simulink model "DHM"  (R2022a)
settings: Solver=FixedStepDiscrete  StartTime=0.0  StopTime=10.0  FixedStep=0.01  RelTol=1e-3
libraries: simulink x8, DoorHndDriver x4, DoorHndReq x4, DoorHndPosSts x4
(part 1 of 2)
settings Model: Creator=DELL  LastModifiedBy=DELL
settings DataIOCC: SaveFormat=StructureWithTime
settings OptimizationCC: DefaultParameterBehavior=Inlined  EnhancedBackFolding=on  PassReuseOutputArgsAs=Individual arguments  ZeroExternalMemoryAtStartup=off  ZeroInternalMemoryAtStartup=off  OptimizeBlockOrder=speed  DifferentSizesBufferReuse=on  OptimizationCustomize=off  EfficientTunableParamExpr=on
settings DebuggingCC: ParameterTunabilityLossMsg=error
settings ModelReferenceCC: ModelReferenceNumInstancesAllowed=Single
settings SFSimCC: MATLABDynamicMemAlloc=off
settings RTWCC: Description=AUTOSAR  SystemTargetFile=autosar.tlc  GenCodeOnly=on  TemplateMakefile=ert_default_tmf
settings CodeAppCC: ForceParamTrailComments=on  IgnoreCustomStorageClasses=off  OperatorAnnotations=on  SimulinkDataObjDesc=on  SFDataObjDesc=on  InsertBlockDesc=on
settings STFCustomTargetCC: TargetLangStandard=C99 (ISO)  MultiwordLength=256  ParMdlRefBuildCompliant=on  CompOptLevelCompliant=on  IncludeMdlTerminateFcn=off  CombineOutputUpdateFcns=on  SuppressErrorStatus=on  ERTCustomFileBanners=on  SupportNonFinite=off  SupportComplex=off  SupportContinuousTime=off  SupportNonInlinedSFcns=off  RemoveResetFunc=on  MATLABClassNameForMDSCustomization=Simulink.SoftwareTarget.ERTCustomization  AutosarCompliant=on  GRTInterface=off  UseToolchainInfoCompliant=on  LookupTableObjectStructAxisOrder=2,1,3,4,...  LUTObjectStructOrderEvenSpacing=Size,Table,Breakpoints  SystemTargetFile=autosar.tlc
settings ERTTargetCC: TargetLangStandard=C99 (ISO)  ConcurrentExecutionCompliant=off  IncludeMdlTerminateFcn=off  SuppressErrorStatus=on  SupportNonFinite=off  SupportComplex=off  ModelStepFunctionPrototypeControlCompliant=off  CPPClassGenCompliant=off  AutosarCompliant=on  LookupTableObjectStructAxisOrder=2,1,3,4,...  LUTObjectStructOrderEvenSpacing=Size,Table,Breakpoints  InlinedParameterPlacement=NonHierarchical  ERTCustomFileTemplate=example_file_process.tlc

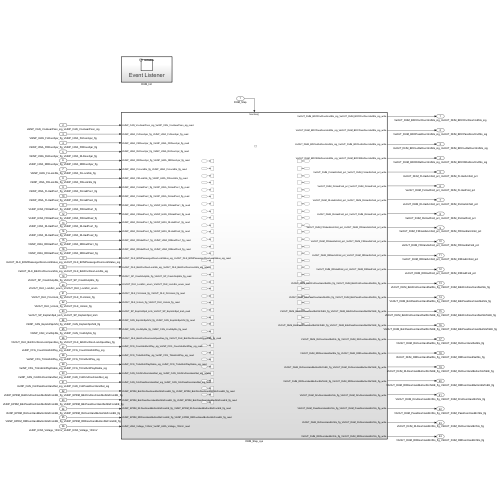
[thumbnail: Simulink's stored preview of the top-level diagram]
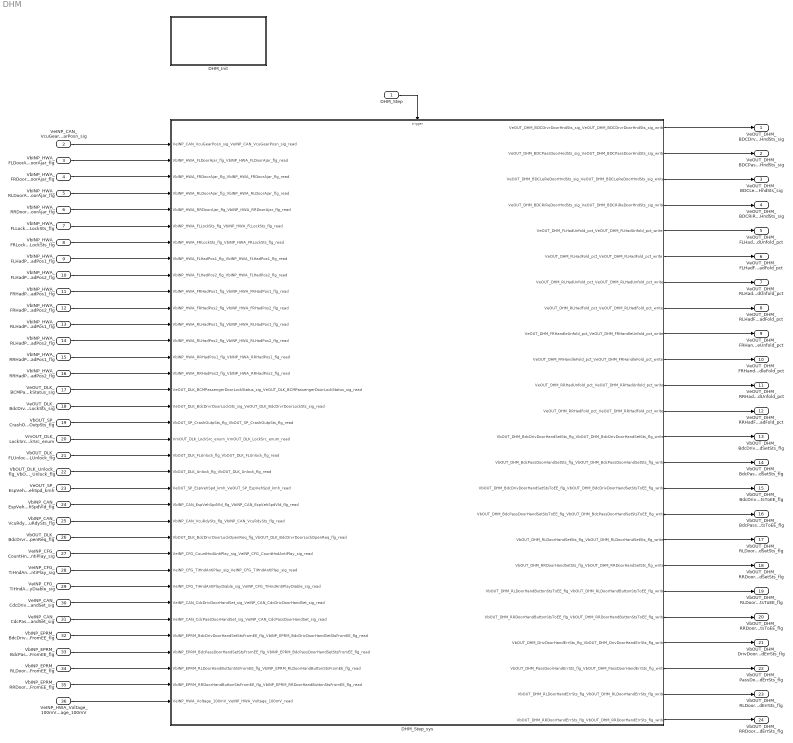
== system DHM ==
  DHM_Step : Inport  SampleTime=0.01  OutputFunctionCall=on
  VeINP_CAN_VcuGearPosn_sig_VeINP_CAN_VcuGearPosn_sig : Inport  Port=2  OutDataTypeStr=UInt8  PortDimensions=1
  VbINP_HWA_FLDoorAjar_flg_VbINP_HWA_FLDoorAjar_flg : Inport  Port=3  OutDataTypeStr=Boolean  PortDimensions=1
  VbINP_HWA_FRDoorAjar_flg_VbINP_HWA_FRDoorAjar_flg : Inport  Port=4  OutDataTypeStr=Boolean  PortDimensions=1
  VbINP_HWA_RLDoorAjar_flg_VbINP_HWA_RLDoorAjar_flg : Inport  Port=5  OutDataTypeStr=Boolean  PortDimensions=1
  VbINP_HWA_RRDoorAjar_flg_VbINP_HWA_RRDoorAjar_flg : Inport  Port=6  OutDataTypeStr=Boolean  PortDimensions=1
  VbINP_HWA_FLLockSts_flg_VbINP_HWA_FLLockSts_flg : Inport  Port=7  OutDataTypeStr=Boolean  PortDimensions=1
  VbINP_HWA_FRLockSts_flg_VbINP_HWA_FRLockSts_flg : Inport  Port=8  OutDataTypeStr=Boolean  PortDimensions=1
  VbINP_HWA_FLHadPos1_flg_VbINP_HWA_FLHadPos1_flg : Inport  Port=9  OutDataTypeStr=Boolean  PortDimensions=1
  VbINP_HWA_FLHadPos2_flg_VbINP_HWA_FLHadPos2_flg : Inport  Port=10  OutDataTypeStr=Boolean  PortDimensions=1
  VbINP_HWA_FRHadPos1_flg_VbINP_HWA_FRHadPos1_flg : Inport  Port=11  OutDataTypeStr=Boolean  PortDimensions=1
  VbINP_HWA_FRHadPos2_flg_VbINP_HWA_FRHadPos2_flg : Inport  Port=12  OutDataTypeStr=Boolean  PortDimensions=1
  VbINP_HWA_RLHadPos1_flg_VbINP_HWA_RLHadPos1_flg : Inport  Port=13  OutDataTypeStr=Boolean  PortDimensions=1
  VbINP_HWA_RLHadPos2_flg_VbINP_HWA_RLHadPos2_flg : Inport  Port=14  OutDataTypeStr=Boolean  PortDimensions=1
  VbINP_HWA_RRHadPos1_flg_VbINP_HWA_RRHadPos1_flg : Inport  Port=15  OutDataTypeStr=Boolean  PortDimensions=1
  VbINP_HWA_RRHadPos2_flg_VbINP_HWA_RRHadPos2_flg : Inport  Port=16  OutDataTypeStr=Boolean  PortDimensions=1
  VeOUT_DLK_BCMPassengerDoorLockStatus_sig_VeOUT_DLK_BCMPassengerDoorLockStatus_sig : Inport  Port=17  OutDataTypeStr=UInt8  PortDimensions=1
  VeOUT_DLK_BdcDrvrDoorLockSts_sig_VeOUT_DLK_BdcDrvrDoorLockSts_sig : Inport  Port=18  OutDataTypeStr=UInt8  PortDimensions=1
  VbOUT_SP_CrashOutpSts_flg_VbOUT_SP_CrashOutpSts_flg : Inport  Port=19  OutDataTypeStr=Boolean  PortDimensions=1
  VmOUT_DLK_LockSrc_enum_VmOUT_DLK_LockSrc_enum : Inport  Port=20  OutDataTypeStr=UInt8  PortDimensions=1
  VbOUT_DLK_FLUnlock_flg_VbOUT_DLK_FLUnlock_flg : Inport  Port=21  OutDataTypeStr=Boolean  PortDimensions=1
  VbOUT_DLK_Unlock_flg_VbOUT_DLK_Unlock_flg : Inport  Port=22  OutDataTypeStr=Boolean  PortDimensions=1
  VeOUT_SP_EspVehSpd_kmh_VeOUT_SP_EspVehSpd_kmh : Inport  Port=23  OutDataTypeStr=UInt8  PortDimensions=1
  VbINP_CAN_EspVehSpdVld_flg_VbINP_CAN_EspVehSpdVld_flg : Inport  Port=24  OutDataTypeStr=Boolean  PortDimensions=1
  VbINP_CAN_VcuRdySts_flg_VbINP_CAN_VcuRdySts_flg : Inport  Port=25  OutDataTypeStr=Boolean  PortDimensions=1
  VbOUT_DLK_BdcDrvrDoorLockOpenReq_flg_VbOUT_DLK_BdcDrvrDoorLockOpenReq_flg : Inport  Port=26  OutDataTypeStr=Boolean  PortDimensions=1
  VeINP_CFG_CountHndAntiPlay_sig_VeINP_CFG_CountHndAntiPlay_sig : Inport  Port=27  OutDataTypeStr=UInt8  PortDimensions=1
  VeINP_CFG_TiHndAntiPlay_sig_VeINP_CFG_TiHndAntiPlay_sig : Inport  Port=28  OutDataTypeStr=UInt8  PortDimensions=1
  VeINP_CFG_TiHndAntiPlayDiable_sig_VeINP_CFG_TiHndAntiPlayDiable_sig : Inport  Port=29  OutDataTypeStr=UInt8  PortDimensions=1
  VeINP_CAN_CdcDrivDoorHandSet_sig_VeINP_CAN_CdcDrivDoorHandSet_sig : Inport  Port=30  OutDataTypeStr=UInt8  PortDimensions=1
  VeINP_CAN_CdcPassDoorHandSet_sig_VeINP_CAN_CdcPassDoorHandSet_sig : Inport  Port=31  OutDataTypeStr=UInt8  PortDimensions=1
  VbINP_EPRM_BdcDrivDoorHandSetStsFromEE_flg_VbINP_EPRM_BdcDrivDoorHandSetStsFromEE_flg : Inport  Port=32  OutDataTypeStr=Boolean  PortDimensions=1
  VbINP_EPRM_BdcPassDoorHandSetStsFromEE_flg_VbINP_EPRM_BdcPassDoorHandSetStsFromEE_flg : Inport  Port=33  OutDataTypeStr=Boolean  PortDimensions=1
  VbINP_EPRM_RLDoorHandButtonStsFromEE_flg_VbINP_EPRM_RLDoorHandButtonStsFromEE_flg : Inport  Port=34  OutDataTypeStr=Boolean  PortDimensions=1
  VbINP_EPRM_RRDoorHandButtonStsFromEE_flg_VbINP_EPRM_RRDoorHandButtonStsFromEE_flg : Inport  Port=35  OutDataTypeStr=Boolean  PortDimensions=1
  VeINP_HWA_Voltage_100mV_VeINP_HWA_Voltage_100mV : Inport  Port=36  OutDataTypeStr=UInt8  PortDimensions=1
  DHM_Init : Subsystem
  DHM_Step_sys : Subsystem
  VeOUT_DHM_BDCDrvrDoorHndSts_sig_VeOUT_DHM_BDCDrvrDoorHndSts_sig : Outport  OutDataTypeStr=UInt8  PortDimensions=1
  VeOUT_DHM_BDCPassDoorHndSts_sig_VeOUT_DHM_BDCPassDoorHndSts_sig : Outport  Port=2  OutDataTypeStr=UInt8  PortDimensions=1
  VeOUT_DHM_BDCLeReDoorHndSts_sig_VeOUT_DHM_BDCLeReDoorHndSts_sig : Outport  Port=3  OutDataTypeStr=UInt8  PortDimensions=1
  VeOUT_DHM_BDCRiReDoorHndSts_sig_VeOUT_DHM_BDCRiReDoorHndSts_sig : Outport  Port=4  OutDataTypeStr=UInt8  PortDimensions=1
  VeOUT_DHM_FLHadUnfold_pct_VeOUT_DHM_FLHadUnfold_pct : Outport  Port=5  OutDataTypeStr=UInt8  PortDimensions=1
  VeOUT_DHM_FLHadFold_pct_VeOUT_DHM_FLHadFold_pct : Outport  Port=6  OutDataTypeStr=UInt8  PortDimensions=1
  VeOUT_DHM_RLHadUnfold_pct_VeOUT_DHM_RLHadUnfold_pct : Outport  Port=7  OutDataTypeStr=UInt8  PortDimensions=1
  VeOUT_DHM_RLHadFold_pct_VeOUT_DHM_RLHadFold_pct : Outport  Port=8  OutDataTypeStr=UInt8  PortDimensions=1
  VeOUT_DHM_FRHandleUnfold_pct_VeOUT_DHM_FRHandleUnfold_pct : Outport  Port=9  OutDataTypeStr=UInt8  PortDimensions=1
  VeOUT_DHM_FRHandleFold_pct_VeOUT_DHM_FRHandleFold_pct : Outport  Port=10  OutDataTypeStr=UInt8  PortDimensions=1
  VeOUT_DHM_RRHadUnfold_pct_VeOUT_DHM_RRHadUnfold_pct : Outport  Port=11  OutDataTypeStr=UInt8  PortDimensions=1
  VeOUT_DHM_RRHadFold_pct_VeOUT_DHM_RRHadFold_pct : Outport  Port=12  OutDataTypeStr=UInt8  PortDimensions=1
  VbOUT_DHM_BdcDrivDoorHandSetSts_flg_VbOUT_DHM_BdcDrivDoorHandSetSts_flg : Outport  Port=13  OutDataTypeStr=Boolean  PortDimensions=1
  VbOUT_DHM_BdcPassDoorHandSetSts_flg_VbOUT_DHM_BdcPassDoorHandSetSts_flg : Outport  Port=14  OutDataTypeStr=Boolean  PortDimensions=1
  VbOUT_DHM_BdcDrivDoorHandSetStsToEE_flg_VbOUT_DHM_BdcDrivDoorHandSetStsToEE_flg : Outport  Port=15  OutDataTypeStr=Boolean  PortDimensions=1
  VbOUT_DHM_BdcPassDoorHandSetStsToEE_flg_VbOUT_DHM_BdcPassDoorHandSetStsToEE_flg : Outport  Port=16  OutDataTypeStr=Boolean  PortDimensions=1
  VbOUT_DHM_RLDoorHandSetSts_flg_VbOUT_DHM_RLDoorHandSetSts_flg : Outport  Port=17  OutDataTypeStr=Boolean  PortDimensions=1
  VbOUT_DHM_RRDoorHandSetSts_flg_VbOUT_DHM_RRDoorHandSetSts_flg : Outport  Port=18  OutDataTypeStr=Boolean  PortDimensions=1
  VbOUT_DHM_RLDoorHandButtonStsToEE_flg_VbOUT_DHM_RLDoorHandButtonStsToEE_flg : Outport  Port=19  OutDataTypeStr=Boolean  PortDimensions=1
  VbOUT_DHM_RRDoorHandButtonStsToEE_flg_VbOUT_DHM_RRDoorHandButtonStsToEE_flg : Outport  Port=20  OutDataTypeStr=Boolean  PortDimensions=1
  VbOUT_DHM_DrivDoorHandErrSts_flg_VbOUT_DHM_DrivDoorHandErrSts_flg : Outport  Port=21  OutDataTypeStr=Boolean  PortDimensions=1
  VbOUT_DHM_PassDoorHandErrSts_flg_VbOUT_DHM_PassDoorHandErrSts_flg : Outport  Port=22  OutDataTypeStr=Boolean  PortDimensions=1
  VbOUT_DHM_RLDoorHandErrSts_flg_VbOUT_DHM_RLDoorHandErrSts_flg : Outport  Port=23  OutDataTypeStr=Boolean  PortDimensions=1
  VbOUT_DHM_RRDoorHandErrSts_flg_VbOUT_DHM_RRDoorHandErrSts_flg : Outport  Port=24  OutDataTypeStr=Boolean  PortDimensions=1
  wires:
  VeINP_CAN_VcuGearPosn_sig_VeINP_CAN_VcuGearPosn_sig/1 -> DHM_Step_sys/1(VeINP_CAN_VcuGearPosn_sig_VeINP_CAN_VcuGearPosn_sig_read)
  VbINP_HWA_FLDoorAjar_flg_VbINP_HWA_FLDoorAjar_flg/1 -> DHM_Step_sys/2(VbINP_HWA_FLDoorAjar_flg_VbINP_HWA_FLDoorAjar_flg_read)
  VbINP_HWA_FRDoorAjar_flg_VbINP_HWA_FRDoorAjar_flg/1 -> DHM_Step_sys/3(VbINP_HWA_FRDoorAjar_flg_VbINP_HWA_FRDoorAjar_flg_read)
  VbINP_HWA_RLDoorAjar_flg_VbINP_HWA_RLDoorAjar_flg/1 -> DHM_Step_sys/4(VbINP_HWA_RLDoorAjar_flg_VbINP_HWA_RLDoorAjar_flg_read)
  VbINP_HWA_RRDoorAjar_flg_VbINP_HWA_RRDoorAjar_flg/1 -> DHM_Step_sys/5(VbINP_HWA_RRDoorAjar_flg_VbINP_HWA_RRDoorAjar_flg_read)
  VbINP_HWA_FLLockSts_flg_VbINP_HWA_FLLockSts_flg/1 -> DHM_Step_sys/6(VbINP_HWA_FLLockSts_flg_VbINP_HWA_FLLockSts_flg_read)
  VbINP_HWA_FRLockSts_flg_VbINP_HWA_FRLockSts_flg/1 -> DHM_Step_sys/7(VbINP_HWA_FRLockSts_flg_VbINP_HWA_FRLockSts_flg_read)
  VbINP_HWA_FLHadPos1_flg_VbINP_HWA_FLHadPos1_flg/1 -> DHM_Step_sys/8(VbINP_HWA_FLHadPos1_flg_VbINP_HWA_FLHadPos1_flg_read)
  VbINP_HWA_FLHadPos2_flg_VbINP_HWA_FLHadPos2_flg/1 -> DHM_Step_sys/9(VbINP_HWA_FLHadPos2_flg_VbINP_HWA_FLHadPos2_flg_read)
  VbINP_HWA_FRHadPos1_flg_VbINP_HWA_FRHadPos1_flg/1 -> DHM_Step_sys/10(VbINP_HWA_FRHadPos1_flg_VbINP_HWA_FRHadPos1_flg_read)
  VbINP_HWA_FRHadPos2_flg_VbINP_HWA_FRHadPos2_flg/1 -> DHM_Step_sys/11(VbINP_HWA_FRHadPos2_flg_VbINP_HWA_FRHadPos2_flg_read)
  VbINP_HWA_RLHadPos1_flg_VbINP_HWA_RLHadPos1_flg/1 -> DHM_Step_sys/12(VbINP_HWA_RLHadPos1_flg_VbINP_HWA_RLHadPos1_flg_read)
  VbINP_HWA_RLHadPos2_flg_VbINP_HWA_RLHadPos2_flg/1 -> DHM_Step_sys/13(VbINP_HWA_RLHadPos2_flg_VbINP_HWA_RLHadPos2_flg_read)
  VbINP_HWA_RRHadPos1_flg_VbINP_HWA_RRHadPos1_flg/1 -> DHM_Step_sys/14(VbINP_HWA_RRHadPos1_flg_VbINP_HWA_RRHadPos1_flg_read)
  VbINP_HWA_RRHadPos2_flg_VbINP_HWA_RRHadPos2_flg/1 -> DHM_Step_sys/15(VbINP_HWA_RRHadPos2_flg_VbINP_HWA_RRHadPos2_flg_read)
  VeOUT_DLK_BCMPassengerDoorLockStatus_sig_VeOUT_DLK_BCMPassengerDoorLockStatus_sig/1 -> DHM_Step_sys/16(VeOUT_DLK_BCMPassengerDoorLockStatus_sig_VeOUT_DLK_BCMPassengerDoorLockStatus_sig_read)
  VeOUT_DLK_BdcDrvrDoorLockSts_sig_VeOUT_DLK_BdcDrvrDoorLockSts_sig/1 -> DHM_Step_sys/17(VeOUT_DLK_BdcDrvrDoorLockSts_sig_VeOUT_DLK_BdcDrvrDoorLockSts_sig_read)
  VbOUT_SP_CrashOutpSts_flg_VbOUT_SP_CrashOutpSts_flg/1 -> DHM_Step_sys/18(VbOUT_SP_CrashOutpSts_flg_VbOUT_SP_CrashOutpSts_flg_read)
  VmOUT_DLK_LockSrc_enum_VmOUT_DLK_LockSrc_enum/1 -> DHM_Step_sys/19(VmOUT_DLK_LockSrc_enum_VmOUT_DLK_LockSrc_enum_read)
  VbOUT_DLK_FLUnlock_flg_VbOUT_DLK_FLUnlock_flg/1 -> DHM_Step_sys/20(VbOUT_DLK_FLUnlock_flg_VbOUT_DLK_FLUnlock_flg_read)
  VbOUT_DLK_Unlock_flg_VbOUT_DLK_Unlock_flg/1 -> DHM_Step_sys/21(VbOUT_DLK_Unlock_flg_VbOUT_DLK_Unlock_flg_read)
  VeOUT_SP_EspVehSpd_kmh_VeOUT_SP_EspVehSpd_kmh/1 -> DHM_Step_sys/22(VeOUT_SP_EspVehSpd_kmh_VeOUT_SP_EspVehSpd_kmh_read)
  VbINP_CAN_EspVehSpdVld_flg_VbINP_CAN_EspVehSpdVld_flg/1 -> DHM_Step_sys/23(VbINP_CAN_EspVehSpdVld_flg_VbINP_CAN_EspVehSpdVld_flg_read)
  VbINP_CAN_VcuRdySts_flg_VbINP_CAN_VcuRdySts_flg/1 -> DHM_Step_sys/24(VbINP_CAN_VcuRdySts_flg_VbINP_CAN_VcuRdySts_flg_read)
  VbOUT_DLK_BdcDrvrDoorLockOpenReq_flg_VbOUT_DLK_BdcDrvrDoorLockOpenReq_flg/1 -> DHM_Step_sys/25(VbOUT_DLK_BdcDrvrDoorLockOpenReq_flg_VbOUT_DLK_BdcDrvrDoorLockOpenReq_flg_read)
  VeINP_CFG_CountHndAntiPlay_sig_VeINP_CFG_CountHndAntiPlay_sig/1 -> DHM_Step_sys/26(VeINP_CFG_CountHndAntiPlay_sig_VeINP_CFG_CountHndAntiPlay_sig_read)
  VeINP_CFG_TiHndAntiPlay_sig_VeINP_CFG_TiHndAntiPlay_sig/1 -> DHM_Step_sys/27(VeINP_CFG_TiHndAntiPlay_sig_VeINP_CFG_TiHndAntiPlay_sig_read)
  VeINP_CFG_TiHndAntiPlayDiable_sig_VeINP_CFG_TiHndAntiPlayDiable_sig/1 -> DHM_Step_sys/28(VeINP_CFG_TiHndAntiPlayDiable_sig_VeINP_CFG_TiHndAntiPlayDiable_sig_read)
  VeINP_CAN_CdcDrivDoorHandSet_sig_VeINP_CAN_CdcDrivDoorHandSet_sig/1 -> DHM_Step_sys/29(VeINP_CAN_CdcDrivDoorHandSet_sig_VeINP_CAN_CdcDrivDoorHandSet_sig_read)
  VeINP_CAN_CdcPassDoorHandSet_sig_VeINP_CAN_CdcPassDoorHandSet_sig/1 -> DHM_Step_sys/30(VeINP_CAN_CdcPassDoorHandSet_sig_VeINP_CAN_CdcPassDoorHandSet_sig_read)
  VbINP_EPRM_BdcDrivDoorHandSetStsFromEE_flg_VbINP_EPRM_BdcDrivDoorHandSetStsFromEE_flg/1 -> DHM_Step_sys/31(VbINP_EPRM_BdcDrivDoorHandSetStsFromEE_flg_VbINP_EPRM_BdcDrivDoorHandSetStsFromEE_flg_read)
  VbINP_EPRM_BdcPassDoorHandSetStsFromEE_flg_VbINP_EPRM_BdcPassDoorHandSetStsFromEE_flg/1 -> DHM_Step_sys/32(VbINP_EPRM_BdcPassDoorHandSetStsFromEE_flg_VbINP_EPRM_BdcPassDoorHandSetStsFromEE_flg_read)
  VbINP_EPRM_RLDoorHandButtonStsFromEE_flg_VbINP_EPRM_RLDoorHandButtonStsFromEE_flg/1 -> DHM_Step_sys/33(VbINP_EPRM_RLDoorHandButtonStsFromEE_flg_VbINP_EPRM_RLDoorHandButtonStsFromEE_flg_read)
  VbINP_EPRM_RRDoorHandButtonStsFromEE_flg_VbINP_EPRM_RRDoorHandButtonStsFromEE_flg/1 -> DHM_Step_sys/34(VbINP_EPRM_RRDoorHandButtonStsFromEE_flg_VbINP_EPRM_RRDoorHandButtonStsFromEE_flg_read)
  VeINP_HWA_Voltage_100mV_VeINP_HWA_Voltage_100mV/1 -> DHM_Step_sys/35(VeINP_HWA_Voltage_100mV_VeINP_HWA_Voltage_100mV_read)
  DHM_Step_sys/1(VeOUT_DHM_BDCDrvrDoorHndSts_sig_VeOUT_DHM_BDCDrvrDoorHndSts_sig_write) -> VeOUT_DHM_BDCDrvrDoorHndSts_sig_VeOUT_DHM_BDCDrvrDoorHndSts_sig/1
  DHM_Step_sys/2(VeOUT_DHM_BDCPassDoorHndSts_sig_VeOUT_DHM_BDCPassDoorHndSts_sig_write) -> VeOUT_DHM_BDCPassDoorHndSts_sig_VeOUT_DHM_BDCPassDoorHndSts_sig/1
  DHM_Step_sys/3(VeOUT_DHM_BDCLeReDoorHndSts_sig_VeOUT_DHM_BDCLeReDoorHndSts_sig_write) -> VeOUT_DHM_BDCLeReDoorHndSts_sig_VeOUT_DHM_BDCLeReDoorHndSts_sig/1
  DHM_Step_sys/4(VeOUT_DHM_BDCRiReDoorHndSts_sig_VeOUT_DHM_BDCRiReDoorHndSts_sig_write) -> VeOUT_DHM_BDCRiReDoorHndSts_sig_VeOUT_DHM_BDCRiReDoorHndSts_sig/1
  DHM_Step_sys/5(VeOUT_DHM_FLHadUnfold_pct_VeOUT_DHM_FLHadUnfold_pct_write) -> VeOUT_DHM_FLHadUnfold_pct_VeOUT_DHM_FLHadUnfold_pct/1
  DHM_Step_sys/6(VeOUT_DHM_FLHadFold_pct_VeOUT_DHM_FLHadFold_pct_write) -> VeOUT_DHM_FLHadFold_pct_VeOUT_DHM_FLHadFold_pct/1
  DHM_Step_sys/7(VeOUT_DHM_RLHadUnfold_pct_VeOUT_DHM_RLHadUnfold_pct_write) -> VeOUT_DHM_RLHadUnfold_pct_VeOUT_DHM_RLHadUnfold_pct/1
  DHM_Step_sys/8(VeOUT_DHM_RLHadFold_pct_VeOUT_DHM_RLHadFold_pct_write) -> VeOUT_DHM_RLHadFold_pct_VeOUT_DHM_RLHadFold_pct/1
  DHM_Step_sys/9(VeOUT_DHM_FRHandleUnfold_pct_VeOUT_DHM_FRHandleUnfold_pct_write) -> VeOUT_DHM_FRHandleUnfold_pct_VeOUT_DHM_FRHandleUnfold_pct/1
  DHM_Step_sys/10(VeOUT_DHM_FRHandleFold_pct_VeOUT_DHM_FRHandleFold_pct_write) -> VeOUT_DHM_FRHandleFold_pct_VeOUT_DHM_FRHandleFold_pct/1
  DHM_Step_sys/11(VeOUT_DHM_RRHadUnfold_pct_VeOUT_DHM_RRHadUnfold_pct_write) -> VeOUT_DHM_RRHadUnfold_pct_VeOUT_DHM_RRHadUnfold_pct/1
  DHM_Step_sys/12(VeOUT_DHM_RRHadFold_pct_VeOUT_DHM_RRHadFold_pct_write) -> VeOUT_DHM_RRHadFold_pct_VeOUT_DHM_RRHadFold_pct/1
  DHM_Step_sys/13(VbOUT_DHM_BdcDrivDoorHandSetSts_flg_VbOUT_DHM_BdcDrivDoorHandSetSts_flg_write) -> VbOUT_DHM_BdcDrivDoorHandSetSts_flg_VbOUT_DHM_BdcDrivDoorHandSetSts_flg/1
  DHM_Step_sys/14(VbOUT_DHM_BdcPassDoorHandSetSts_flg_VbOUT_DHM_BdcPassDoorHandSetSts_flg_write) -> VbOUT_DHM_BdcPassDoorHandSetSts_flg_VbOUT_DHM_BdcPassDoorHandSetSts_flg/1
  DHM_Step_sys/15(VbOUT_DHM_BdcDrivDoorHandSetStsToEE_flg_VbOUT_DHM_BdcDrivDoorHandSetStsToEE_flg_write) -> VbOUT_DHM_BdcDrivDoorHandSetStsToEE_flg_VbOUT_DHM_BdcDrivDoorHandSetStsToEE_flg/1
  DHM_Step_sys/16(VbOUT_DHM_BdcPassDoorHandSetStsToEE_flg_VbOUT_DHM_BdcPassDoorHandSetStsToEE_flg_write) -> VbOUT_DHM_BdcPassDoorHandSetStsToEE_flg_VbOUT_DHM_BdcPassDoorHandSetStsToEE_flg/1
  DHM_Step_sys/17(VbOUT_DHM_RLDoorHandSetSts_flg_VbOUT_DHM_RLDoorHandSetSts_flg_write) -> VbOUT_DHM_RLDoorHandSetSts_flg_VbOUT_DHM_RLDoorHandSetSts_flg/1
  DHM_Step_sys/18(VbOUT_DHM_RRDoorHandSetSts_flg_VbOUT_DHM_RRDoorHandSetSts_flg_write) -> VbOUT_DHM_RRDoorHandSetSts_flg_VbOUT_DHM_RRDoorHandSetSts_flg/1
  DHM_Step_sys/19(VbOUT_DHM_RLDoorHandButtonStsToEE_flg_VbOUT_DHM_RLDoorHandButtonStsToEE_flg_write) -> VbOUT_DHM_RLDoorHandButtonStsToEE_flg_VbOUT_DHM_RLDoorHandButtonStsToEE_flg/1
  DHM_Step_sys/20(VbOUT_DHM_RRDoorHandButtonStsToEE_flg_VbOUT_DHM_RRDoorHandButtonStsToEE_flg_write) -> VbOUT_DHM_RRDoorHandButtonStsToEE_flg_VbOUT_DHM_RRDoorHandButtonStsToEE_flg/1
  DHM_Step_sys/21(VbOUT_DHM_DrivDoorHandErrSts_flg_VbOUT_DHM_DrivDoorHandErrSts_flg_write) -> VbOUT_DHM_DrivDoorHandErrSts_flg_VbOUT_DHM_DrivDoorHandErrSts_flg/1
  DHM_Step_sys/22(VbOUT_DHM_PassDoorHandErrSts_flg_VbOUT_DHM_PassDoorHandErrSts_flg_write) -> VbOUT_DHM_PassDoorHandErrSts_flg_VbOUT_DHM_PassDoorHandErrSts_flg/1
  DHM_Step_sys/23(VbOUT_DHM_RLDoorHandErrSts_flg_VbOUT_DHM_RLDoorHandErrSts_flg_write) -> VbOUT_DHM_RLDoorHandErrSts_flg_VbOUT_DHM_RLDoorHandErrSts_flg/1
  DHM_Step_sys/24(VbOUT_DHM_RRDoorHandErrSts_flg_VbOUT_DHM_RRDoorHandErrSts_flg_write) -> VbOUT_DHM_RRDoorHandErrSts_flg_VbOUT_DHM_RRDoorHandErrSts_flg/1
  DHM_Step/1 -> DHM_Step_sys/Trigger

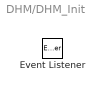
== system DHM/DHM_Init ==
  Event Listener : EventListener  EventName=reset

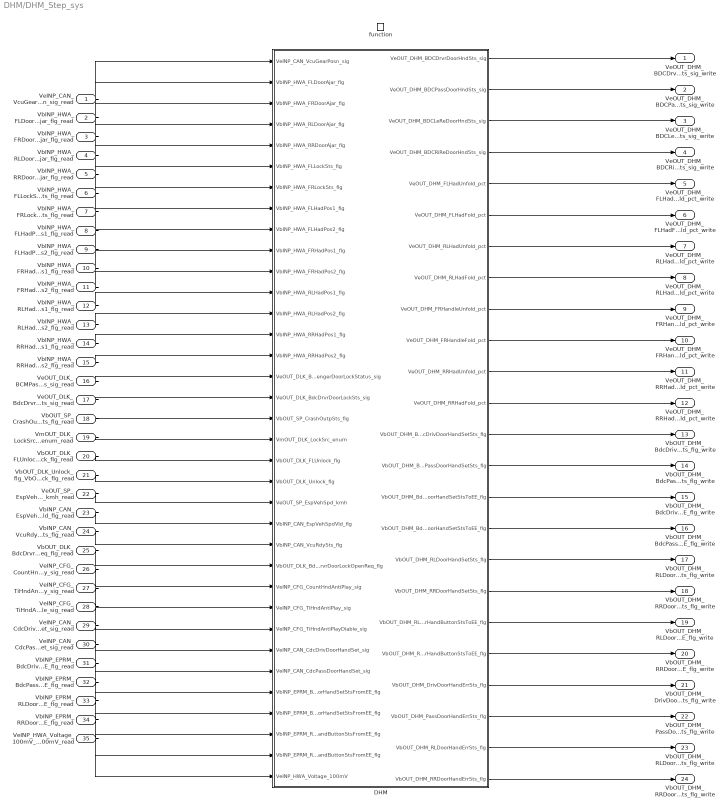
== system DHM/DHM_Step_sys ==
  VeINP_CAN_VcuGearPosn_sig_VeINP_CAN_VcuGearPosn_sig_read : Inport
  VbINP_HWA_FLDoorAjar_flg_VbINP_HWA_FLDoorAjar_flg_read : Inport  Port=2
  VbINP_HWA_FRDoorAjar_flg_VbINP_HWA_FRDoorAjar_flg_read : Inport  Port=3
  VbINP_HWA_RLDoorAjar_flg_VbINP_HWA_RLDoorAjar_flg_read : Inport  Port=4
  VbINP_HWA_RRDoorAjar_flg_VbINP_HWA_RRDoorAjar_flg_read : Inport  Port=5
  VbINP_HWA_FLLockSts_flg_VbINP_HWA_FLLockSts_flg_read : Inport  Port=6
  VbINP_HWA_FRLockSts_flg_VbINP_HWA_FRLockSts_flg_read : Inport  Port=7
  VbINP_HWA_FLHadPos1_flg_VbINP_HWA_FLHadPos1_flg_read : Inport  Port=8
  VbINP_HWA_FLHadPos2_flg_VbINP_HWA_FLHadPos2_flg_read : Inport  Port=9
  VbINP_HWA_FRHadPos1_flg_VbINP_HWA_FRHadPos1_flg_read : Inport  Port=10
  VbINP_HWA_FRHadPos2_flg_VbINP_HWA_FRHadPos2_flg_read : Inport  Port=11
  VbINP_HWA_RLHadPos1_flg_VbINP_HWA_RLHadPos1_flg_read : Inport  Port=12
  VbINP_HWA_RLHadPos2_flg_VbINP_HWA_RLHadPos2_flg_read : Inport  Port=13
  VbINP_HWA_RRHadPos1_flg_VbINP_HWA_RRHadPos1_flg_read : Inport  Port=14
  VbINP_HWA_RRHadPos2_flg_VbINP_HWA_RRHadPos2_flg_read : Inport  Port=15
  VeOUT_DLK_BCMPassengerDoorLockStatus_sig_VeOUT_DLK_BCMPassengerDoorLockStatus_sig_read : Inport  Port=16
  VeOUT_DLK_BdcDrvrDoorLockSts_sig_VeOUT_DLK_BdcDrvrDoorLockSts_sig_read : Inport  Port=17
  VbOUT_SP_CrashOutpSts_flg_VbOUT_SP_CrashOutpSts_flg_read : Inport  Port=18
  VmOUT_DLK_LockSrc_enum_VmOUT_DLK_LockSrc_enum_read : Inport  Port=19
  VbOUT_DLK_FLUnlock_flg_VbOUT_DLK_FLUnlock_flg_read : Inport  Port=20
  VbOUT_DLK_Unlock_flg_VbOUT_DLK_Unlock_flg_read : Inport  Port=21
  VeOUT_SP_EspVehSpd_kmh_VeOUT_SP_EspVehSpd_kmh_read : Inport  Port=22
  VbINP_CAN_EspVehSpdVld_flg_VbINP_CAN_EspVehSpdVld_flg_read : Inport  Port=23
  VbINP_CAN_VcuRdySts_flg_VbINP_CAN_VcuRdySts_flg_read : Inport  Port=24
  VbOUT_DLK_BdcDrvrDoorLockOpenReq_flg_VbOUT_DLK_BdcDrvrDoorLockOpenReq_flg_read : Inport  Port=25
  VeINP_CFG_CountHndAntiPlay_sig_VeINP_CFG_CountHndAntiPlay_sig_read : Inport  Port=26
  VeINP_CFG_TiHndAntiPlay_sig_VeINP_CFG_TiHndAntiPlay_sig_read : Inport  Port=27
  VeINP_CFG_TiHndAntiPlayDiable_sig_VeINP_CFG_TiHndAntiPlayDiable_sig_read : Inport  Port=28
  VeINP_CAN_CdcDrivDoorHandSet_sig_VeINP_CAN_CdcDrivDoorHandSet_sig_read : Inport  Port=29
  VeINP_CAN_CdcPassDoorHandSet_sig_VeINP_CAN_CdcPassDoorHandSet_sig_read : Inport  Port=30
  VbINP_EPRM_BdcDrivDoorHandSetStsFromEE_flg_VbINP_EPRM_BdcDrivDoorHandSetStsFromEE_flg_read : Inport  Port=31
  VbINP_EPRM_BdcPassDoorHandSetStsFromEE_flg_VbINP_EPRM_BdcPassDoorHandSetStsFromEE_flg_read : Inport  Port=32
  VbINP_EPRM_RLDoorHandButtonStsFromEE_flg_VbINP_EPRM_RLDoorHandButtonStsFromEE_flg_read : Inport  Port=33
  VbINP_EPRM_RRDoorHandButtonStsFromEE_flg_VbINP_EPRM_RRDoorHandButtonStsFromEE_flg_read : Inport  Port=34
  VeINP_HWA_Voltage_100mV_VeINP_HWA_Voltage_100mV_read : Inport  Port=35
  function : TriggerPort  TriggerType=function-call  VariantControl=(inherit)  SampleTimeType=periodic  SampleTime=-1
  DHM : Subsystem
  VeOUT_DHM_BDCDrvrDoorHndSts_sig_VeOUT_DHM_BDCDrvrDoorHndSts_sig_write : Outport
      settings: EnsureOutportIsVirtual=on
  VeOUT_DHM_BDCPassDoorHndSts_sig_VeOUT_DHM_BDCPassDoorHndSts_sig_write : Outport  Port=2
      settings: EnsureOutportIsVirtual=on
  VeOUT_DHM_BDCLeReDoorHndSts_sig_VeOUT_DHM_BDCLeReDoorHndSts_sig_write : Outport  Port=3
      settings: EnsureOutportIsVirtual=on
  VeOUT_DHM_BDCRiReDoorHndSts_sig_VeOUT_DHM_BDCRiReDoorHndSts_sig_write : Outport  Port=4
      settings: EnsureOutportIsVirtual=on
  VeOUT_DHM_FLHadUnfold_pct_VeOUT_DHM_FLHadUnfold_pct_write : Outport  Port=5
      settings: EnsureOutportIsVirtual=on
  VeOUT_DHM_FLHadFold_pct_VeOUT_DHM_FLHadFold_pct_write : Outport  Port=6
      settings: EnsureOutportIsVirtual=on
  VeOUT_DHM_RLHadUnfold_pct_VeOUT_DHM_RLHadUnfold_pct_write : Outport  Port=7
      settings: EnsureOutportIsVirtual=on
  VeOUT_DHM_RLHadFold_pct_VeOUT_DHM_RLHadFold_pct_write : Outport  Port=8
      settings: EnsureOutportIsVirtual=on
  VeOUT_DHM_FRHandleUnfold_pct_VeOUT_DHM_FRHandleUnfold_pct_write : Outport  Port=9
      settings: EnsureOutportIsVirtual=on
  VeOUT_DHM_FRHandleFold_pct_VeOUT_DHM_FRHandleFold_pct_write : Outport  Port=10
      settings: EnsureOutportIsVirtual=on
  VeOUT_DHM_RRHadUnfold_pct_VeOUT_DHM_RRHadUnfold_pct_write : Outport  Port=11
      settings: EnsureOutportIsVirtual=on
  VeOUT_DHM_RRHadFold_pct_VeOUT_DHM_RRHadFold_pct_write : Outport  Port=12
      settings: EnsureOutportIsVirtual=on
  VbOUT_DHM_BdcDrivDoorHandSetSts_flg_VbOUT_DHM_BdcDrivDoorHandSetSts_flg_write : Outport  Port=13
      settings: EnsureOutportIsVirtual=on
  VbOUT_DHM_BdcPassDoorHandSetSts_flg_VbOUT_DHM_BdcPassDoorHandSetSts_flg_write : Outport  Port=14
      settings: EnsureOutportIsVirtual=on
  VbOUT_DHM_BdcDrivDoorHandSetStsToEE_flg_VbOUT_DHM_BdcDrivDoorHandSetStsToEE_flg_write : Outport  Port=15
      settings: EnsureOutportIsVirtual=on
  VbOUT_DHM_BdcPassDoorHandSetStsToEE_flg_VbOUT_DHM_BdcPassDoorHandSetStsToEE_flg_write : Outport  Port=16
      settings: EnsureOutportIsVirtual=on
  VbOUT_DHM_RLDoorHandSetSts_flg_VbOUT_DHM_RLDoorHandSetSts_flg_write : Outport  Port=17
      settings: EnsureOutportIsVirtual=on
  VbOUT_DHM_RRDoorHandSetSts_flg_VbOUT_DHM_RRDoorHandSetSts_flg_write : Outport  Port=18
      settings: EnsureOutportIsVirtual=on
  VbOUT_DHM_RLDoorHandButtonStsToEE_flg_VbOUT_DHM_RLDoorHandButtonStsToEE_flg_write : Outport  Port=19
      settings: EnsureOutportIsVirtual=on
  VbOUT_DHM_RRDoorHandButtonStsToEE_flg_VbOUT_DHM_RRDoorHandButtonStsToEE_flg_write : Outport  Port=20
      settings: EnsureOutportIsVirtual=on
  VbOUT_DHM_DrivDoorHandErrSts_flg_VbOUT_DHM_DrivDoorHandErrSts_flg_write : Outport  Port=21
      settings: EnsureOutportIsVirtual=on
  VbOUT_DHM_PassDoorHandErrSts_flg_VbOUT_DHM_PassDoorHandErrSts_flg_write : Outport  Port=22
      settings: EnsureOutportIsVirtual=on
  VbOUT_DHM_RLDoorHandErrSts_flg_VbOUT_DHM_RLDoorHandErrSts_flg_write : Outport  Port=23
      settings: EnsureOutportIsVirtual=on
  VbOUT_DHM_RRDoorHandErrSts_flg_VbOUT_DHM_RRDoorHandErrSts_flg_write : Outport  Port=24
      settings: EnsureOutportIsVirtual=on
  wires:
  DHM/4(VeOUT_DHM_BDCRiReDoorHndSts_sig) -> VeOUT_DHM_BDCRiReDoorHndSts_sig_VeOUT_DHM_BDCRiReDoorHndSts_sig_write/1
  DHM/3(VeOUT_DHM_BDCLeReDoorHndSts_sig) -> VeOUT_DHM_BDCLeReDoorHndSts_sig_VeOUT_DHM_BDCLeReDoorHndSts_sig_write/1
  DHM/5(VeOUT_DHM_FLHadUnfold_pct) -> VeOUT_DHM_FLHadUnfold_pct_VeOUT_DHM_FLHadUnfold_pct_write/1
  DHM/2(VeOUT_DHM_BDCPassDoorHndSts_sig) -> VeOUT_DHM_BDCPassDoorHndSts_sig_VeOUT_DHM_BDCPassDoorHndSts_sig_write/1
  DHM/1(VeOUT_DHM_BDCDrvrDoorHndSts_sig) -> VeOUT_DHM_BDCDrvrDoorHndSts_sig_VeOUT_DHM_BDCDrvrDoorHndSts_sig_write/1
  DHM/6(VeOUT_DHM_FLHadFold_pct) -> VeOUT_DHM_FLHadFold_pct_VeOUT_DHM_FLHadFold_pct_write/1
  DHM/7(VeOUT_DHM_RLHadUnfold_pct) -> VeOUT_DHM_RLHadUnfold_pct_VeOUT_DHM_RLHadUnfold_pct_write/1
  DHM/8(VeOUT_DHM_RLHadFold_pct) -> VeOUT_DHM_RLHadFold_pct_VeOUT_DHM_RLHadFold_pct_write/1
  DHM/9(VeOUT_DHM_FRHandleUnfold_pct) -> VeOUT_DHM_FRHandleUnfold_pct_VeOUT_DHM_FRHandleUnfold_pct_write/1
  DHM/10(VeOUT_DHM_FRHandleFold_pct) -> VeOUT_DHM_FRHandleFold_pct_VeOUT_DHM_FRHandleFold_pct_write/1
  DHM/11(VeOUT_DHM_RRHadUnfold_pct) -> VeOUT_DHM_RRHadUnfold_pct_VeOUT_DHM_RRHadUnfold_pct_write/1
  DHM/12(VeOUT_DHM_RRHadFold_pct) -> VeOUT_DHM_RRHadFold_pct_VeOUT_DHM_RRHadFold_pct_write/1
  DHM/13(VbOUT_DHM_BdcDrivDoorHandSetSts_flg) -> VbOUT_DHM_BdcDrivDoorHandSetSts_flg_VbOUT_DHM_BdcDrivDoorHandSetSts_flg_write/1
  DHM/14(VbOUT_DHM_BdcPassDoorHandSetSts_flg) -> VbOUT_DHM_BdcPassDoorHandSetSts_flg_VbOUT_DHM_BdcPassDoorHandSetSts_flg_write/1
  DHM/15(VbOUT_DHM_BdcDrivDoorHandSetStsToEE_flg) -> VbOUT_DHM_BdcDrivDoorHandSetStsToEE_flg_VbOUT_DHM_BdcDrivDoorHandSetStsToEE_flg_write/1
  DHM/16(VbOUT_DHM_BdcPassDoorHandSetStsToEE_flg) -> VbOUT_DHM_BdcPassDoorHandSetStsToEE_flg_VbOUT_DHM_BdcPassDoorHandSetStsToEE_flg_write/1
  DHM/17("VbOUT_DHM_RLDoorHandSetSts_flg ") -> VbOUT_DHM_RLDoorHandSetSts_flg_VbOUT_DHM_RLDoorHandSetSts_flg_write/1
  DHM/18("VbOUT_DHM_RRDoorHandSetSts_flg ") -> VbOUT_DHM_RRDoorHandSetSts_flg_VbOUT_DHM_RRDoorHandSetSts_flg_write/1
  DHM/19("VbOUT_DHM_RLDoorHandButtonStsToEE_flg ") -> VbOUT_DHM_RLDoorHandButtonStsToEE_flg_VbOUT_DHM_RLDoorHandButtonStsToEE_flg_write/1
  DHM/20("VbOUT_DHM_RRDoorHandButtonStsToEE_flg ") -> VbOUT_DHM_RRDoorHandButtonStsToEE_flg_VbOUT_DHM_RRDoorHandButtonStsToEE_flg_write/1
  DHM/21(VbOUT_DHM_DrivDoorHandErrSts_flg) -> VbOUT_DHM_DrivDoorHandErrSts_flg_VbOUT_DHM_DrivDoorHandErrSts_flg_write/1
  DHM/22(VbOUT_DHM_PassDoorHandErrSts_flg) -> VbOUT_DHM_PassDoorHandErrSts_flg_VbOUT_DHM_PassDoorHandErrSts_flg_write/1
  DHM/23(VbOUT_DHM_RLDoorHandErrSts_flg) -> VbOUT_DHM_RLDoorHandErrSts_flg_VbOUT_DHM_RLDoorHandErrSts_flg_write/1
  DHM/24(VbOUT_DHM_RRDoorHandErrSts_flg) -> VbOUT_DHM_RRDoorHandErrSts_flg_VbOUT_DHM_RRDoorHandErrSts_flg_write/1
  VbINP_HWA_RRDoorAjar_flg_VbINP_HWA_RRDoorAjar_flg_read/1 -> DHM/5(VbINP_HWA_RRDoorAjar_flg)
  VbINP_HWA_FLLockSts_flg_VbINP_HWA_FLLockSts_flg_read/1 -> DHM/6(VbINP_HWA_FLLockSts_flg)
  VbINP_HWA_RLDoorAjar_flg_VbINP_HWA_RLDoorAjar_flg_read/1 -> DHM/4(VbINP_HWA_RLDoorAjar_flg)
  VbINP_HWA_FRDoorAjar_flg_VbINP_HWA_FRDoorAjar_flg_read/1 -> DHM/3(VbINP_HWA_FRDoorAjar_flg)
  VbINP_HWA_FRLockSts_flg_VbINP_HWA_FRLockSts_flg_read/1 -> DHM/7(VbINP_HWA_FRLockSts_flg)
  VbINP_HWA_FLDoorAjar_flg_VbINP_HWA_FLDoorAjar_flg_read/1 -> DHM/2(VbINP_HWA_FLDoorAjar_flg)
  VbINP_HWA_FLHadPos1_flg_VbINP_HWA_FLHadPos1_flg_read/1 -> DHM/8(VbINP_HWA_FLHadPos1_flg)
  VbINP_HWA_FLHadPos2_flg_VbINP_HWA_FLHadPos2_flg_read/1 -> DHM/9(VbINP_HWA_FLHadPos2_flg)
  VeINP_CAN_VcuGearPosn_sig_VeINP_CAN_VcuGearPosn_sig_read/1 -> DHM/1(VeINP_CAN_VcuGearPosn_sig)
  VbINP_HWA_FRHadPos1_flg_VbINP_HWA_FRHadPos1_flg_read/1 -> DHM/10(VbINP_HWA_FRHadPos1_flg)
  VbINP_HWA_FRHadPos2_flg_VbINP_HWA_FRHadPos2_flg_read/1 -> DHM/11(VbINP_HWA_FRHadPos2_flg)
  VbINP_HWA_RLHadPos1_flg_VbINP_HWA_RLHadPos1_flg_read/1 -> DHM/12(VbINP_HWA_RLHadPos1_flg)
  VbINP_HWA_RLHadPos2_flg_VbINP_HWA_RLHadPos2_flg_read/1 -> DHM/13(VbINP_HWA_RLHadPos2_flg)
  VbINP_HWA_RRHadPos1_flg_VbINP_HWA_RRHadPos1_flg_read/1 -> DHM/14(VbINP_HWA_RRHadPos1_flg)
  VbINP_HWA_RRHadPos2_flg_VbINP_HWA_RRHadPos2_flg_read/1 -> DHM/15(VbINP_HWA_RRHadPos2_flg)
  VeOUT_DLK_BCMPassengerDoorLockStatus_sig_VeOUT_DLK_BCMPassengerDoorLockStatus_sig_read/1 -> DHM/16(VeOUT_DLK_BCMPassengerDoorLockStatus_sig)
  VeOUT_DLK_BdcDrvrDoorLockSts_sig_VeOUT_DLK_BdcDrvrDoorLockSts_sig_read/1 -> DHM/17(VeOUT_DLK_BdcDrvrDoorLockSts_sig)
  VbOUT_SP_CrashOutpSts_flg_VbOUT_SP_CrashOutpSts_flg_read/1 -> DHM/18(VbOUT_SP_CrashOutpSts_flg)
  VmOUT_DLK_LockSrc_enum_VmOUT_DLK_LockSrc_enum_read/1 -> DHM/19(VmOUT_DLK_LockSrc_enum)
  VbOUT_DLK_FLUnlock_flg_VbOUT_DLK_FLUnlock_flg_read/1 -> DHM/20(VbOUT_DLK_FLUnlock_flg)
  VbOUT_DLK_Unlock_flg_VbOUT_DLK_Unlock_flg_read/1 -> DHM/21(VbOUT_DLK_Unlock_flg)
  VeOUT_SP_EspVehSpd_kmh_VeOUT_SP_EspVehSpd_kmh_read/1 -> DHM/22(VeOUT_SP_EspVehSpd_kmh)
  VbINP_CAN_EspVehSpdVld_flg_VbINP_CAN_EspVehSpdVld_flg_read/1 -> DHM/23(VbINP_CAN_EspVehSpdVld_flg)
  VbINP_CAN_VcuRdySts_flg_VbINP_CAN_VcuRdySts_flg_read/1 -> DHM/24(VbINP_CAN_VcuRdySts_flg)
  VbOUT_DLK_BdcDrvrDoorLockOpenReq_flg_VbOUT_DLK_BdcDrvrDoorLockOpenReq_flg_read/1 -> DHM/25(VbOUT_DLK_BdcDrvrDoorLockOpenReq_flg)
  VeINP_CFG_CountHndAntiPlay_sig_VeINP_CFG_CountHndAntiPlay_sig_read/1 -> DHM/26(VeINP_CFG_CountHndAntiPlay_sig)
  VeINP_CFG_TiHndAntiPlay_sig_VeINP_CFG_TiHndAntiPlay_sig_read/1 -> DHM/27(VeINP_CFG_TiHndAntiPlay_sig)
  VeINP_CFG_TiHndAntiPlayDiable_sig_VeINP_CFG_TiHndAntiPlayDiable_sig_read/1 -> DHM/28(VeINP_CFG_TiHndAntiPlayDiable_sig)
  VeINP_CAN_CdcDrivDoorHandSet_sig_VeINP_CAN_CdcDrivDoorHandSet_sig_read/1 -> DHM/29(VeINP_CAN_CdcDrivDoorHandSet_sig)
  VeINP_CAN_CdcPassDoorHandSet_sig_VeINP_CAN_CdcPassDoorHandSet_sig_read/1 -> DHM/30(VeINP_CAN_CdcPassDoorHandSet_sig)
  VbINP_EPRM_BdcDrivDoorHandSetStsFromEE_flg_VbINP_EPRM_BdcDrivDoorHandSetStsFromEE_flg_read/1 -> DHM/31(VbINP_EPRM_BdcDrivDoorHandSetStsFromEE_flg)
  VbINP_EPRM_BdcPassDoorHandSetStsFromEE_flg_VbINP_EPRM_BdcPassDoorHandSetStsFromEE_flg_read/1 -> DHM/32(VbINP_EPRM_BdcPassDoorHandSetStsFromEE_flg)
  VbINP_EPRM_RLDoorHandButtonStsFromEE_flg_VbINP_EPRM_RLDoorHandButtonStsFromEE_flg_read/1 -> DHM/33(VbINP_EPRM_RLDoorHandButtonStsFromEE_flg)
  VbINP_EPRM_RRDoorHandButtonStsFromEE_flg_VbINP_EPRM_RRDoorHandButtonStsFromEE_flg_read/1 -> DHM/34(VbINP_EPRM_RRDoorHandButtonStsFromEE_flg)
  VeINP_HWA_Voltage_100mV_VeINP_HWA_Voltage_100mV_read/1 -> DHM/35(VeINP_HWA_Voltage_100mV)

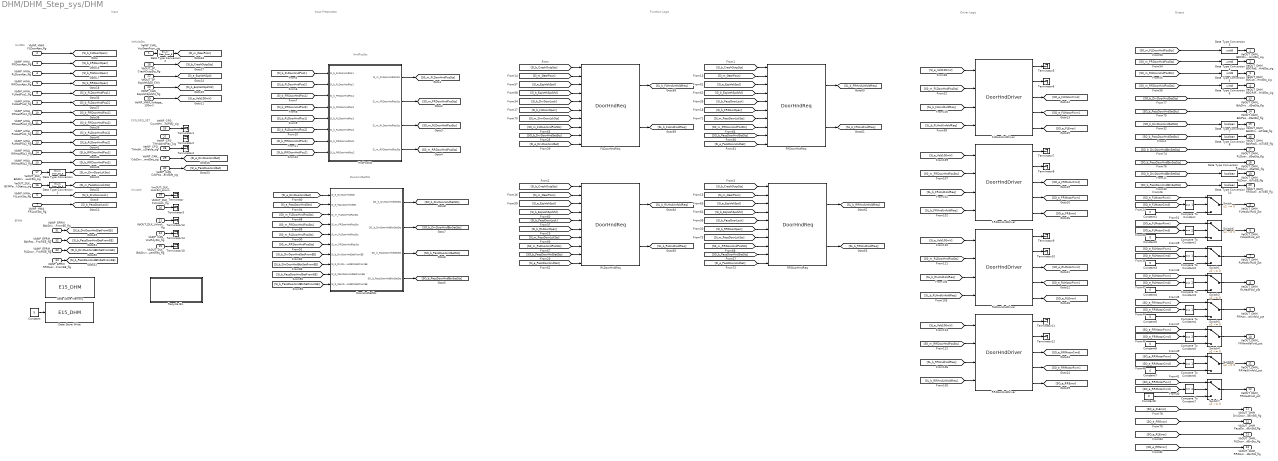
== system DHM/DHM_Step_sys/DHM ==
  note: HndSts
  note: Output
  note: Driver Logic
  note: Function Logic
  note: Input Preprocess
  note: Input
  note: VehicleSts
  note: Unused
  note: CFG_REQ_SET
  note: EPRM
  note: HndPosSts
  note: DoorHndSetSts
  VeINP_CAN_VcuGearPosn_sig : Inport
  VbINP_HWA_FLDoorAjar_flg : Inport  Port=2
  VbINP_HWA_FRDoorAjar_flg : Inport  Port=3
  VbINP_HWA_RLDoorAjar_flg : Inport  Port=4
  VbINP_HWA_RRDoorAjar_flg : Inport  Port=5
  VbINP_HWA_FLLockSts_flg : Inport  Port=6
  VbINP_HWA_FRLockSts_flg : Inport  Port=7
  VbINP_HWA_FLHadPos1_flg : Inport  Port=8
  VbINP_HWA_FLHadPos2_flg : Inport  Port=9
  VbINP_HWA_FRHadPos1_flg : Inport  Port=10
  VbINP_HWA_FRHadPos2_flg : Inport  Port=11
  VbINP_HWA_RLHadPos1_flg : Inport  Port=12
  VbINP_HWA_RLHadPos2_flg : Inport  Port=13
  VbINP_HWA_RRHadPos1_flg : Inport  Port=14
  VbINP_HWA_RRHadPos2_flg : Inport  Port=15
  VeOUT_DLK_BCMPassengerDoorLockStatus_sig : Inport  Port=16
  VeOUT_DLK_BdcDrvrDoorLockSts_sig : Inport  Port=17
  VbOUT_SP_CrashOutpSts_flg : Inport  Port=18
  VmOUT_DLK_LockSrc_enum : Inport  Port=19
  VbOUT_DLK_FLUnlock_flg : Inport  Port=20
  VbOUT_DLK_Unlock_flg : Inport  Port=21
  VeOUT_SP_EspVehSpd_kmh : Inport  Port=22
  VbINP_CAN_EspVehSpdVld_flg : Inport  Port=23
  VbINP_CAN_VcuRdySts_flg : Inport  Port=24
  VbOUT_DLK_BdcDrvrDoorLockOpenReq_flg : Inport  Port=25
  VeINP_CFG_CountHndAntiPlay_sig : Inport  Port=26
  VeINP_CFG_TiHndAntiPlay_sig : Inport  Port=27
  VeINP_CFG_TiHndAntiPlayDiable_sig : Inport  Port=28
  VeINP_CAN_CdcDrivDoorHandSet_sig : Inport  Port=29
  VeINP_CAN_CdcPassDoorHandSet_sig : Inport  Port=30
  VbINP_EPRM_BdcDrivDoorHandSetStsFromEE_flg : Inport  Port=31
  VbINP_EPRM_BdcPassDoorHandSetStsFromEE_flg : Inport  Port=32
  VbINP_EPRM_RLDoorHandButtonStsFromEE_flg : Inport  Port=33
  VbINP_EPRM_RRDoorHandButtonStsFromEE_flg : Inport  Port=34
  VeINP_HWA_Voltage_100mV : Inport  Port=35
  Compare To Constant{,2,4,6} (4 alike) : simulink/Logic and Bit Operations/Compare To Constant  relop===  const=1  OutDataTypeStr=boolean
  Compare To Constant{1,3,5,7} (4 alike) : simulink/Logic and Bit Operations/Compare To Constant  relop===  const=2  OutDataTypeStr=boolean
  Constant : Constant  Value=5  OutDataTypeStr=uint8
  Constant{1..8} (8 alike) : Constant  Value=0
  Data Store Memory : DataStoreMemory  DataStoreName=E15_DHM  WriteAfterWriteMsg=warning  ShowAdditionalParam=off  OutDataTypeStr=uint8
  Data Store Write : DataStoreWrite  DataStoreName=E15_DHM  IndexOptions=Index vector (dialog)  Indices=1  OutputSizes=1
  Data Type Conversion : DataTypeConversion  OutDataTypeStr=Enum: Door_Sts_E  SaturateOnIntegerOverflow=off  RndMeth=Floor
  Data Type Conversion1 : DataTypeConversion  OutDataTypeStr=Enum: Door_Sts_E  SaturateOnIntegerOverflow=off  RndMeth=Floor
  Data Type Conversion{7..10} (4 alike) : DataTypeConversion  OutDataTypeStr=boolean  SaturateOnIntegerOverflow=off  RndMeth=Floor
  Data Type Conversion2 : DataTypeConversion  OutDataTypeStr=Enum: Gear_Posn_E  SaturateOnIntegerOverflow=off  RndMeth=Floor
  Data Type Conversion{3..6} (4 alike) : DataTypeConversion  OutDataTypeStr=uint8  SaturateOnIntegerOverflow=off  RndMeth=Floor
  DoorHndSetSts : Stateflow chart  TreatAsAtomicUnit=on
  FLDoorHndDriver : DoorHndDriver/DoorHndDriver  SystemSampleTime=-1  VariantActivationTime=update diagram  Latency=0  AutoFrameSizeCalculation=off
  FLDoorHndReq : DoorHndReq/DoorHndReq  SystemSampleTime=-1  VariantActivationTime=update diagram  Latency=0  AutoFrameSizeCalculation=off
  FRDoorHndDriver : DoorHndDriver/DoorHndDriver  SystemSampleTime=-1  VariantActivationTime=update diagram  Latency=0  AutoFrameSizeCalculation=off
  FRDoorHndReq : DoorHndReq/DoorHndReq  SystemSampleTime=-1  VariantActivationTime=update diagram  Latency=0  AutoFrameSizeCalculation=off
  HndPosSts : Stateflow chart  TreatAsAtomicUnit=on
  RLDoorHndDriver : DoorHndDriver/DoorHndDriver  SystemSampleTime=-1  VariantActivationTime=update diagram  Latency=0  AutoFrameSizeCalculation=off
  RLDoorHndReq : DoorHndReq/DoorHndReq  SystemSampleTime=-1  VariantActivationTime=update diagram  Latency=0  AutoFrameSizeCalculation=off
  RRDoorHndDriver : DoorHndDriver/DoorHndDriver  SystemSampleTime=-1  VariantActivationTime=update diagram  Latency=0  AutoFrameSizeCalculation=off
  RRDoorHndReq : DoorHndReq/DoorHndReq  SystemSampleTime=-1  VariantActivationTime=update diagram  Latency=0  AutoFrameSizeCalculation=off
  Recycle Bin : Subsystem
  Switch{,1..7} (8 alike) : Switch  Criteria=u2 ~= 0  OutDataTypeStr=uint8  SaturateOnIntegerOverflow=off  InputSameDT=off
  Terminator{,1..14,19} (16 alike) : Terminator
  VeOUT_DHM_BDCDrvrDoorHndSts_sig : Outport
  VeOUT_DHM_BDCPassDoorHndSts_sig : Outport  Port=2
  VeOUT_DHM_BDCLeReDoorHndSts_sig : Outport  Port=3
  VeOUT_DHM_BDCRiReDoorHndSts_sig : Outport  Port=4
  VeOUT_DHM_FLHadUnfold_pct : Outport  Port=5
  VeOUT_DHM_FLHadFold_pct : Outport  Port=6
  VeOUT_DHM_RLHadUnfold_pct : Outport  Port=7
  VeOUT_DHM_RLHadFold_pct : Outport  Port=8
  VeOUT_DHM_FRHandleUnfold_pct : Outport  Port=9
  VeOUT_DHM_FRHandleFold_pct : Outport  Port=10
  VeOUT_DHM_RRHadUnfold_pct : Outport  Port=11
  VeOUT_DHM_RRHadFold_pct : Outport  Port=12
  VbOUT_DHM_BdcDrivDoorHandSetSts_flg : Outport  Port=13
  VbOUT_DHM_BdcPassDoorHandSetSts_flg : Outport  Port=14
  VbOUT_DHM_BdcDrivDoorHandSetStsToEE_flg : Outport  Port=15
  VbOUT_DHM_BdcPassDoorHandSetStsToEE_flg : Outport  Port=16
  "VbOUT_DHM_RLDoorHandSetSts_flg " : Outport  Port=17
  "VbOUT_DHM_RRDoorHandSetSts_flg " : Outport  Port=18
  "VbOUT_DHM_RLDoorHandButtonStsToEE_flg " : Outport  Port=19
  "VbOUT_DHM_RRDoorHandButtonStsToEE_flg " : Outport  Port=20
  VbOUT_DHM_DrivDoorHandErrSts_flg : Outport  Port=21
  VbOUT_DHM_PassDoorHandErrSts_flg : Outport  Port=22
  VbOUT_DHM_RLDoorHandErrSts_flg : Outport  Port=23
  VbOUT_DHM_RRDoorHandErrSts_flg : Outport  Port=24
  wires:
  VbINP_HWA_FLDoorAjar_flg/1 -> [SI_b_FLDoorOpen]
  VbINP_HWA_FRDoorAjar_flg/1 -> [SI_b_FRDoorOpen]
  VbINP_HWA_RLDoorAjar_flg/1 -> [SI_b_RLDoorOpen]
  VbINP_HWA_RRDoorAjar_flg/1 -> [SI_b_RRDoorOpen]
  VbOUT_SP_CrashOutpSts_flg/1 -> [SI_b_CrashOutpSts]
  [SI_e_DrvDoorHndSet] -> DoorHndSetSts/1(SI_e_DrvDoorHndSet)
  [SI_b_DrvDoorHndBtnSetFromEE] -> DoorHndSetSts/8(SI_b_DrvDoorHndBtnSetFromEE)
  [SI_b_DrvDoorHndSetFromEE] -> DoorHndSetSts/7(SI_b_DrvDoorHndSetFromEE)
  [SI_b_PassDoorHndSetFromEE] -> DoorHndSetSts/9(SI_b_PassDoorHndSetFromEE)
  [SI_b_PassDoorHndBtnSetFromEE] -> DoorHndSetSts/10(SI_b_PassDoorHndBtnSetFromEE)
  [SI_e_PassDoorHndSet] -> DoorHndSetSts/2(SI_e_PassDoorHndSet)
  RLDoorHndReq/1 -> [SL_b_RLHndUnfoldReq]
  RLDoorHndReq/2 -> [SL_b_RLHndFoldReq]
  RRDoorHndReq/2 -> [SL_b_RRHndFoldReq]
  VbINP_HWA_FRHadPos1_flg/1 -> [SI_b_FRDoorHndPos1]
  VbINP_HWA_FRHadPos2_flg/1 -> [SI_b_FRDoorHndPos2]
  VbINP_HWA_RLHadPos1_flg/1 -> [SI_b_RLDoorHndPos1]
  VbINP_HWA_RLHadPos2_flg/1 -> [SI_b_RLDoorHndPos2]
  VbINP_HWA_RRHadPos1_flg/1 -> [SI_b_RRDoorHndPos1]
  VbINP_HWA_RRHadPos2_flg/1 -> [SI_b_RRDoorHndPos2]
  FLDoorHndReq/1 -> [SL_b_FLHndUnfoldReq]
  FLDoorHndReq/2 -> [SL_b_FLHndFoldReq]
  FRDoorHndReq/1 -> [SL_b_FRHndUnfoldReq]
  FRDoorHndReq/2 -> [SL_b_FRHndFoldReq]
  [S0_m_FLDoorHndPosSts] -> FLDoorHndDriver/2
  [SL_b_FLHndUnfoldReq] -> FLDoorHndDriver/4
  [SI_e_Volt100mV] -> FLDoorHndDriver/1
  [SL_b_FLHndFoldReq] -> FLDoorHndDriver/3
  [SI_e_Volt100mV] -> FRDoorHndDriver/1
  [S0_m_FRDoorHndPosSts] -> FRDoorHndDriver/2
  [SI_e_Volt100mV] -> RLDoorHndDriver/1
  [S0_m_RLDoorHndPosSts] -> RLDoorHndDriver/2
  [SI_e_Volt100mV] -> RRDoorHndDriver/1
  [S0_m_RRDoorHndPosSts] -> RRDoorHndDriver/2
  FLDoorHndDriver/1 -> Terminator5/1
  FLDoorHndDriver/2 -> Terminator6/1
  FRDoorHndDriver/1 -> Terminator7/1
  FRDoorHndDriver/2 -> Terminator8/1
  RLDoorHndDriver/1 -> Terminator9/1
  RLDoorHndDriver/2 -> Terminator10/1
  RRDoorHndDriver/1 -> Terminator11/1
  RRDoorHndDriver/2 -> Terminator12/1
  VbINP_HWA_FLHadPos1_flg/1 -> [SI_b_FLDoorHndPos1]
  VbINP_HWA_FLHadPos2_flg/1 -> [SI_b_FLDoorHndPos2]
  VmOUT_DLK_LockSrc_enum/1 -> Terminator/1
  VeOUT_SP_EspVehSpd_kmh/1 -> [SI_e_EspVehSpd]
  VbINP_CAN_EspVehSpdVld_flg/1 -> [SI_b_EspVehSpdVld]
  VeINP_CFG_CountHndAntiPlay_sig/1 -> Terminator1/1
  ? -> Terminator2/1
  VeINP_HWA_Voltage_100mV/1 -> [SI_e_Volt100mV]
  VeINP_CAN_CdcDrivDoorHandSet_sig/1 -> [SI_e_DrvDoorHndSet]
  VeINP_CAN_CdcPassDoorHandSet_sig/1 -> [SI_e_PassDoorHndSet]
  VbOUT_DLK_FLUnlock_flg/1 -> Terminator3/1
  VeOUT_DLK_BCMPassengerDoorLockStatus_sig/1 -> Data Type Conversion1/1
  VeINP_CFG_TiHndAntiPlayDiable_sig/1 -> Terminator4/1
  VbOUT_DLK_Unlock_flg/1 -> Terminator13/1
  VbINP_CAN_VcuRdySts_flg/1 -> Terminator14/1
  Constant/1 -> Data Store Write/1
  RRDoorHndReq/1 -> [SL_b_RRHndUnfoldReq]
  [SI_b_FLDoorHndPos1] -> HndPosSts/1(SI_b_FLDoorHndPos1)
  [SI_b_FLDoorHndPos2] -> HndPosSts/2(SI_b_FLDoorHndPos2)
  [SI_b_FRDoorHndPos1] -> HndPosSts/3(SI_b_FRDoorHndPos1)
  [SI_b_FRDoorHndPos2] -> HndPosSts/4(SI_b_FRDoorHndPos2)
  [SI_b_RLDoorHndPos1] -> HndPosSts/5(SI_b_RLDoorHndPos1)
  [SI_b_RLDoorHndPos2] -> HndPosSts/6(SI_b_RLDoorHndPos2)
  [SI_b_RRDoorHndPos1] -> HndPosSts/7(SI_b_RRDoorHndPos1)
  [SI_b_RRDoorHndPos2] -> HndPosSts/8(SI_b_RRDoorHndPos2)
  HndPosSts/1(SI_m_FLDoorHndPosSts) -> [S0_m_FLDoorHndPosSts]
  HndPosSts/2(SI_m_FRDoorHndPosSts) -> [S0_m_FRDoorHndPosSts]
  HndPosSts/3(SI_m_RLDoorHndPosSts) -> [S0_m_RLDoorHndPosSts]
  HndPosSts/4(SI_m_RRDoorHndPosSts) -> [S0_m_RRDoorHndPosSts]
  [S0_m_RLDoorHndPosSts] -> DoorHndSetSts/5(SI_m_RLDoorHndPosSts)
  [S0_m_FRDoorHndPosSts] -> DoorHndSetSts/4(SI_m_FRDoorHndPosSts)
  [S0_m_RRDoorHndPosSts] -> DoorHndSetSts/6(SI_m_RRDoorHndPosSts)
  [S0_m_FLDoorHndPosSts] -> DoorHndSetSts/3(SI_m_FLDoorHndPosSts)
  Data Type Conversion/1 -> [SI_m_DrvrDoorLckSts]
  Data Type Conversion1/1 -> [SI_m_PassDoorLckSts]
  DoorHndSetSts/1(SO_b_DrvDoorHndSetSts) -> [SO_b_DrvDoorHndSetSts]
  DoorHndSetSts/2(SO_b_DrvDoorHndBtnSetSts) -> [SO_b_DrvDoorHndBtnSetSts]
  DoorHndSetSts/3(SO_b_PassDoorHndSetSts) -> [SO_b_PassDoorHndSetSts]
  DoorHndSetSts/4(SO_b_PassDoorHndBtnSetSts) -> [SO_b_PassDoorHndBtnSetSts]
  VeOUT_DLK_BdcDrvrDoorLockSts_sig/1 -> Data Type Conversion/1
  VbINP_HWA_FLLockSts_flg/1 -> [SI_b_DrvDoorLock]
  VbINP_HWA_FRLockSts_flg/1 -> [SI_b_PassDoorLock]
  [SI_b_CrashOutpSts] -> FLDoorHndReq/1
  [SI_m_GearPosn] -> FLDoorHndReq/2
  [SI_e_EspVehSpd] -> FLDoorHndReq/3
  [SI_b_EspVehSpdVld] -> FLDoorHndReq/4
  [SI_b_DrvDoorLock] -> FLDoorHndReq/5
  [SI_b_FLDoorOpen] -> FLDoorHndReq/6
  [SI_m_DrvrDoorLckSts] -> FLDoorHndReq/7
  [S0_m_FLDoorHndPosSts] -> FLDoorHndReq/8
  [SO_b_DrvDoorHndSetSts] -> FLDoorHndReq/9
  [SI_b_CrashOutpSts] -> FRDoorHndReq/1
  [SI_e_EspVehSpd] -> FRDoorHndReq/3
  [SI_b_PassDoorLock] -> FRDoorHndReq/5
  [SI_b_FRDoorOpen] -> FRDoorHndReq/6
  [SI_m_GearPosn] -> FRDoorHndReq/2
  [SI_b_EspVehSpdVld] -> FRDoorHndReq/4
  [SI_m_PassDoorLckSts] -> FRDoorHndReq/7
  [S0_m_FRDoorHndPosSts] -> FRDoorHndReq/8
  [SO_b_PassDoorHndSetSts] -> FRDoorHndReq/9
  [SI_e_EspVehSpd] -> RLDoorHndReq/3
  [SI_b_EspVehSpdVld] -> RLDoorHndReq/4
  [SI_b_PassDoorLock] -> RLDoorHndReq/5
  [SI_m_GearPosn] -> RLDoorHndReq/2
  [SI_b_RLDoorOpen] -> RLDoorHndReq/6
  [SI_b_CrashOutpSts] -> RLDoorHndReq/1
  [SI_m_PassDoorLckSts] -> RLDoorHndReq/7
  [S0_m_RLDoorHndPosSts] -> RLDoorHndReq/8
  [SO_b_PassDoorHndSetSts] -> RLDoorHndReq/9
  [SI_b_PassDoorLock] -> RRDoorHndReq/5
  [SI_b_CrashOutpSts] -> RRDoorHndReq/1
  [SI_m_PassDoorLckSts] -> RRDoorHndReq/7
  [SI_b_EspVehSpdVld] -> RRDoorHndReq/4
  [SI_b_RRDoorOpen] -> RRDoorHndReq/6
  [S0_m_RRDoorHndPosSts] -> RRDoorHndReq/8
  [SI_e_EspVehSpd] -> RRDoorHndReq/3
  [SO_b_PassDoorHndSetSts] -> RRDoorHndReq/9
  [SI_m_GearPosn] -> RRDoorHndReq/2
  FLDoorHndDriver/3 -> [SO_e_FLMotorCmd]
  FRDoorHndDriver/3 -> [SO_e_FRMotorCmd]
  RLDoorHndDriver/3 -> [SO_e_RLMotorCmd]
  RRDoorHndDriver/3 -> [SO_e_RRMotorCmd]
  [SO_e_FLMotorPwm] -> Switch/1
  [SO_e_FLMotorCmd] -> Compare To Constant/1
  Compare To Constant/1 -> Switch/2
  Constant1/1 -> Switch/3
  [SO_e_FLMotorCmd] -> Compare To Constant1/1
  Compare To Constant1/1 -> Switch6/2
  [SO_e_FLMotorPwm] -> Switch6/1
  Constant2/1 -> Switch6/3
  [SO_e_RLMotorCmd] -> Compare To Constant2/1
  [SO_e_RLMotorPwm] -> Switch1/1
  Compare To Constant2/1 -> Switch1/2
  Constant3/1 -> Switch1/3
  Compare To Constant3/1 -> Switch2/2
  [SO_e_RLMotorCmd] -> Compare To Constant3/1
  [SO_e_RLMotorPwm] -> Switch2/1
  Constant4/1 -> Switch2/3
  Compare To Constant4/1 -> Switch3/2
  [SO_e_FRMotorPwm] -> Switch3/1
  [SO_e_FRMotorCmd] -> Compare To Constant4/1
  Constant5/1 -> Switch3/3
  [SO_e_FRMotorPwm] -> Switch4/1
  [SO_e_FRMotorCmd] -> Compare To Constant5/1
  Compare To Constant5/1 -> Switch4/2
  Constant6/1 -> Switch4/3
  Switch/1 -> VeOUT_DHM_FLHadUnfold_pct/1
  Switch6/1 -> VeOUT_DHM_FLHadFold_pct/1
  Switch1/1 -> VeOUT_DHM_RLHadUnfold_pct/1
  Switch2/1 -> VeOUT_DHM_RLHadFold_pct/1
  Switch3/1 -> VeOUT_DHM_FRHandleUnfold_pct/1
  Switch4/1 -> VeOUT_DHM_FRHandleFold_pct/1
  Switch5/1 -> VeOUT_DHM_RRHadUnfold_pct/1
  [SO_e_RRMotorCmd] -> Compare To Constant6/1
  [SO_e_RRMotorPwm] -> Switch5/1
  Constant7/1 -> Switch5/3
  [SO_e_RRMotorCmd] -> Compare To Constant7/1
  Compare To Constant7/1 -> Switch7/2
  [SO_e_RRMotorPwm] -> Switch7/1
  Constant8/1 -> Switch7/3
  VbOUT_DLK_BdcDrvrDoorLockOpenReq_flg/1 -> Terminator19/1
  VbINP_EPRM_BdcDrivDoorHandSetStsFromEE_flg/1 -> [SI_b_DrvDoorHndSetFromEE]
  VbINP_EPRM_BdcPassDoorHandSetStsFromEE_flg/1 -> [SI_b_PassDoorHndSetFromEE]
  VbINP_EPRM_RLDoorHandButtonStsFromEE_flg/1 -> [SI_b_DrvDoorHndBtnSetFromEE]
  VbINP_EPRM_RRDoorHandButtonStsFromEE_flg/1 -> [SI_b_PassDoorHndBtnSetFromEE]
  VeINP_CAN_VcuGearPosn_sig/1 -> Data Type Conversion2/1
  Data Type Conversion2/1 -> [SI_m_GearPosn]
  Data Type Conversion3/1 -> VeOUT_DHM_BDCDrvrDoorHndSts_sig/1
  Data Type Conversion4/1 -> VeOUT_DHM_BDCPassDoorHndSts_sig/1
  Data Type Conversion5/1 -> VeOUT_DHM_BDCLeReDoorHndSts_sig/1
  Data Type Conversion6/1 -> VeOUT_DHM_BDCRiReDoorHndSts_sig/1
  [S0_m_RRDoorHndPosSts] -> Data Type Conversion6/1
  [S0_m_RLDoorHndPosSts] -> Data Type Conversion5/1
  [S0_m_FRDoorHndPosSts] -> Data Type Conversion4/1
  [S0_m_FLDoorHndPosSts] -> Data Type Conversion3/1
  Switch7/1 -> VeOUT_DHM_RRHadFold_pct/1
  [SI_e_DrvDoorHndSet] -> FLDoorHndReq/10
  [SI_e_PassDoorHndSet] -> FRDoorHndReq/10
  [SI_e_PassDoorHndSet] -> RRDoorHndReq/10
  [SI_e_PassDoorHndSet] -> RLDoorHndReq/10
  FLDoorHndDriver/4 -> [SO_e_FLMotorPwm]
  FLDoorHndDriver/5 -> [SO_e_FLError]
  FRDoorHndDriver/4 -> [SO_e_FRMotorPwm]
  FRDoorHndDriver/5 -> [SO_e_FRError]
  RLDoorHndDriver/4 -> [SO_e_RLMotorPwm]
  RLDoorHndDriver/5 -> [SO_e_RLError]
  RRDoorHndDriver/4 -> [SO_e_RRMotorPwm]
  RRDoorHndDriver/5 -> [SO_e_RRError]
  Compare To Constant6/1 -> Switch5/2
  [SL_b_FRHndFoldReq] -> FRDoorHndDriver/3
  [SL_b_FRHndUnfoldReq] -> FRDoorHndDriver/4
  [SL_b_RLHndFoldReq] -> RLDoorHndDriver/3
  [SL_b_RLHndUnfoldReq] -> RLDoorHndDriver/4
  [SL_b_RRHndFoldReq] -> RRDoorHndDriver/3
  [SL_b_RRHndUnfoldReq] -> RRDoorHndDriver/4
  [SO_b_DrvDoorHndSetSts] -> VbOUT_DHM_BdcDrivDoorHandSetSts_flg/1
  [SO_b_PassDoorHndSetSts] -> VbOUT_DHM_BdcPassDoorHandSetSts_flg/1
  [SO_b_DrvDoorHndBtnSetSts] -> "VbOUT_DHM_RLDoorHandSetSts_flg "/1
  [SO_b_PassDoorHndBtnSetSts] -> "VbOUT_DHM_RRDoorHandSetSts_flg "/1
  [SO_b_DrvDoorHndSetSts] -> Data Type Conversion7/1
  Data Type Conversion7/1 -> VbOUT_DHM_BdcDrivDoorHandSetStsToEE_flg/1
  [SO_b_PassDoorHndSetSts] -> Data Type Conversion8/1
  Data Type Conversion8/1 -> VbOUT_DHM_BdcPassDoorHandSetStsToEE_flg/1
  Data Type Conversion9/1 -> "VbOUT_DHM_RLDoorHandButtonStsToEE_flg "/1
  Data Type Conversion10/1 -> "VbOUT_DHM_RRDoorHandButtonStsToEE_flg "/1
  [SO_b_PassDoorHndBtnSetSts] -> Data Type Conversion10/1
  [SO_b_DrvDoorHndBtnSetSts] -> Data Type Conversion9/1
  [SO_e_FLError] -> VbOUT_DHM_DrivDoorHandErrSts_flg/1
  [SO_e_FRError] -> VbOUT_DHM_PassDoorHandErrSts_flg/1
  [SO_e_RLError] -> VbOUT_DHM_RLDoorHandErrSts_flg/1
  [SO_e_RRError] -> VbOUT_DHM_RRDoorHandErrSts_flg/1

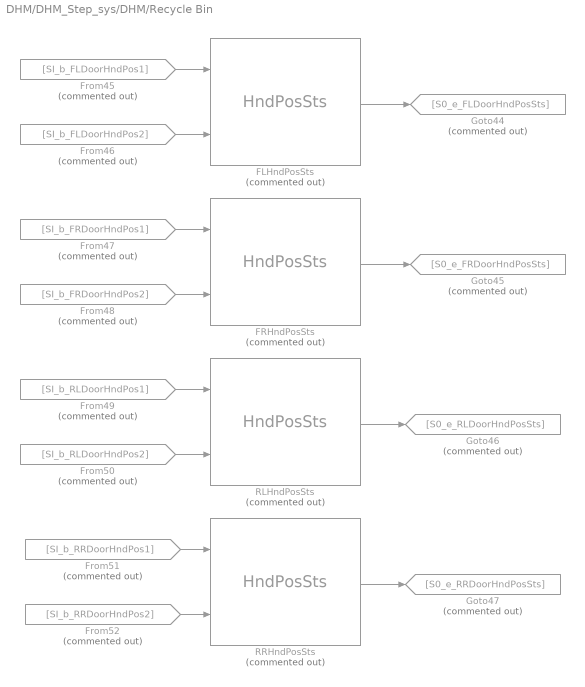
== system DHM/DHM_Step_sys/DHM/Recycle Bin ==
  FLHndPosSts : DoorHndPosSts/HndPosSts  Commented=on  SystemSampleTime=-1  VariantActivationTime=update diagram  Latency=0  AutoFrameSizeCalculation=off
  FRHndPosSts : DoorHndPosSts/HndPosSts  Commented=on  SystemSampleTime=-1  VariantActivationTime=update diagram  Latency=0  AutoFrameSizeCalculation=off
  From45 : From  Commented=on  GotoTag=SI_b_FLDoorHndPos1
  From46 : From  Commented=on  GotoTag=SI_b_FLDoorHndPos2
  From47 : From  Commented=on  GotoTag=SI_b_FRDoorHndPos1
  From48 : From  Commented=on  GotoTag=SI_b_FRDoorHndPos2
  From49 : From  Commented=on  GotoTag=SI_b_RLDoorHndPos1
  From50 : From  Commented=on  GotoTag=SI_b_RLDoorHndPos2
  From51 : From  Commented=on  GotoTag=SI_b_RRDoorHndPos1
  From52 : From  Commented=on  GotoTag=SI_b_RRDoorHndPos2
  Goto44 : Goto  Commented=on  GotoTag=S0_e_FLDoorHndPosSts
  Goto45 : Goto  Commented=on  GotoTag=S0_e_FRDoorHndPosSts
  Goto46 : Goto  Commented=on  GotoTag=S0_e_RLDoorHndPosSts
  Goto47 : Goto  Commented=on  GotoTag=S0_e_RRDoorHndPosSts
  RLHndPosSts : DoorHndPosSts/HndPosSts  Commented=on  SystemSampleTime=-1  VariantActivationTime=update diagram  Latency=0  AutoFrameSizeCalculation=off
  RRHndPosSts : DoorHndPosSts/HndPosSts  Commented=on  SystemSampleTime=-1  VariantActivationTime=update diagram  Latency=0  AutoFrameSizeCalculation=off
  wires:
  From52/1 -> RRHndPosSts/2
  RRHndPosSts/1 -> Goto47/1
  From50/1 -> RLHndPosSts/2
  From45/1 -> FLHndPosSts/1
  From46/1 -> FLHndPosSts/2
  From48/1 -> FRHndPosSts/2
  FLHndPosSts/1 -> Goto44/1
  From47/1 -> FRHndPosSts/1
  From51/1 -> RRHndPosSts/1
  FRHndPosSts/1 -> Goto45/1
  From49/1 -> RLHndPosSts/1
  RLHndPosSts/1 -> Goto46/1
